simulink model "gm_psk_demodulate_block_fil"  (R2020a)
settings: Solver=FixedStepDiscrete  StartTime=0.0  StopTime=10.0  RelTol=1e-3
libraries: simulink x1, hdlmdlgenlib x1, fillib x1
settings Model: Creator=wardo  LastModifiedBy=wardo
settings DataIOCC: LimitDataPoints=on  SaveOutput=off  SaveTime=off
settings OptimizationCC: BlockReduction=off  ConditionallyExecuteInputs=off  DefaultParameterBehavior=Inlined  LifeSpan=inf
settings DebuggingCC: AlgebraicLoopMsg=error  InheritedTsInSrcMsg=none  SingleTaskRateTransMsg=error  AllowSymbolicDim=off  StrictBusMsg=ErrorOnBusTreatedAsVector  SFUnexpectedBacktrackingDiag=warning  SFNoUnconditionalDefaultTransitionDiag=warning  SFExecutionAtInitializationDiag=none  ArithmeticOperatorsInVariantConditions=warning
settings HardwareCC: ProdBitPerPointer=32  ProdBitPerSizeT=32  ProdBitPerPtrDiffT=32  ProdLargestAtomicFloat=None  ProdIntDivRoundTo=Undefined  ProdEndianess=Unspecified  ProdWordSize=32  ProdHWDeviceType=ASIC/FPGA->ASIC/FPGA  ProdEqTarget=off
settings SFSimCC: SimUseLocalCustomCode=off  CustomCodeUndefinedFunction=UseInterfaceOnly
settings RTWCC: RTWUseLocalCustomCode=off
settings CodeAppCC: StateflowObjectComments=on
settings GRTTargetCC: TargetLangStandard=C89/C90 (ANSI)
settings ConfigComp: CovScope=ReferencedModels  CovMetricSettings=dw  CovHtmlReporting=on  CovSaveCumulativeToWorkspaceVar=on  CovSaveSingleToWorkspaceVar=on  CovExternalEMLEnable=off  CovSFcnEnable=off

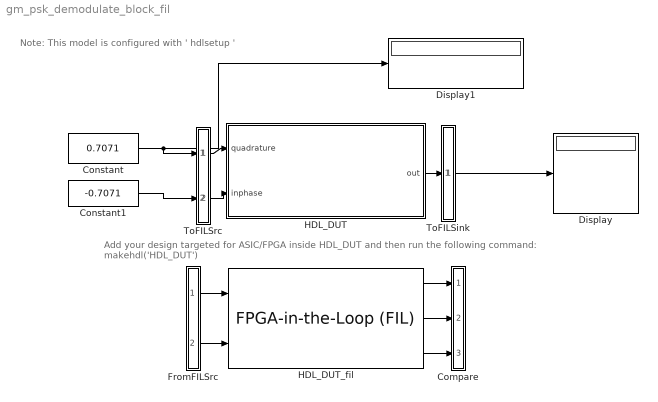
== system gm_psk_demodulate_block_fil ==
  note: Note: This model is configured with ' hdlsetup '
  note: Add your design targeted for ASIC/FPGA inside HDL_DUT and then run the following command:
      | makehdl('HDL_DUT')
  Compare : Subsystem
      mask Display: disp('')
  Constant : Constant  Value=0.7071  OutDataTypeStr=single  SampleTime=-1
  Constant1 : Constant  Value=-0.7071  OutDataTypeStr=single  SampleTime=-1
  Display : Display
  Display1 : Display
  FromFILSrc : Subsystem
      mask Display: disp('')
  HDL_DUT : Subsystem
  HDL_DUT_fil : fillib/FPGA-in-the-Loop (FIL)  ForceInterfaceUpdate=0.90579
      settings: SourceProductBaseCode=ES,HD
  ToFILSink : Subsystem
      mask Display: disp('')
  ToFILSrc : Subsystem
      mask Display: disp('')
  wires:
  Constant/1 -> Display1/1, ToFILSrc/1(in1)
  ToFILSrc/1(out1) -> HDL_DUT/1(quadrature)
  ToFILSrc/2(out2) -> HDL_DUT/2(inphase)
  HDL_DUT/1(out) -> ToFILSink/1(in1)
  Constant1/1 -> ToFILSrc/2(in2)
  ToFILSink/1(out1) -> Display/1
  FromFILSrc/1(out1) -> HDL_DUT_fil/1
  FromFILSrc/2(out2) -> HDL_DUT_fil/2
  HDL_DUT_fil/1 -> Compare/1(in1)
  HDL_DUT_fil/2 -> Compare/2(in2)
  HDL_DUT_fil/3 -> Compare/3(in3)

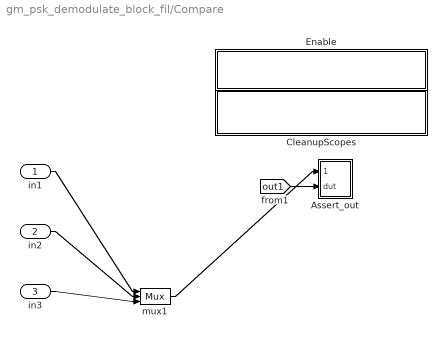
== system gm_psk_demodulate_block_fil/Compare ==
  in1 : Inport
  in2 : Inport  Port=2
  in3 : Inport  Port=3
  Assert_out : Subsystem  mask{ToleranceValue=1e-07}
  CleanupScopes : Subsystem
      settings: OpenFcn=|
      | blkName = gcb; %self block
      | idx = regexp(blkName, '/CleanupScopes$', 'once');
      | blkParent = blkName(1:idx-1);
      | blks=find_system(blkParent, 'LookUnderMasks', 'all','blocktype', 'Scope');
      | for itr = 1:length(blks)
      | 	 hScopeCfg = get_param(blks{itr},'ScopeConfiguration');
      | 	 hScopeCfg.Visible = ~ hScopeCfg.Visible;
      | end
      | drawnow;
      mask Display: fprintf(message('hdlcoder:cosim:vnl_dblclick').getString());
  Enable : Subsystem
      settings: OpenFcn=|
      | blkName = gcb;
      | idx = regexp(blkName, '/Enable$', 'once');
      | blkParent = blkName(1:idx-1);
      | blks=find_system(blkParent, 'LookUnderMasks', 'all','blocktype', 'Assertion');
      | e = get_param(blks{1}, 'Enabled');
      | if strcmp(e, 'on'), f= 'off';, else, f = 'on';, end
      | for ii=1:length(blks), set_param(blks{ii}, 'Enabled', f);, end
      | set_param(gcb, 'MaskDisplay',['fprintf(message(''hdlcoder:cosim:vnl_dblclick_assertions'',','''',upper(e),'''',').getString())']);
      mask Display: fprintf(message('hdlcoder:cosim:vnl_dblclick_assertions','OFF').getString());
  mux1 : Mux  Inputs=3
  wires:
  in3/1 -> mux1/3
  in2/1 -> mux1/2
  in1/1 -> mux1/1
  mux1/1 -> Assert_out/1(cosim)
  [out1] -> Assert_out/2(dut)

== system gm_psk_demodulate_block_fil/FromFILSrc ==
  dtc1 : DataTypeConversion  OutDataTypeStr=single  SaturateOnIntegerOverflow=on  RndMeth=Zero
  dtc2 : DataTypeConversion  OutDataTypeStr=single  SaturateOnIntegerOverflow=on  RndMeth=Zero
  out1 : Outport
  out2 : Outport  Port=2
  wires:
  [in1] -> dtc1/1
  [in2] -> dtc2/1
  dtc1/1 -> out1/1
  dtc2/1 -> out2/1

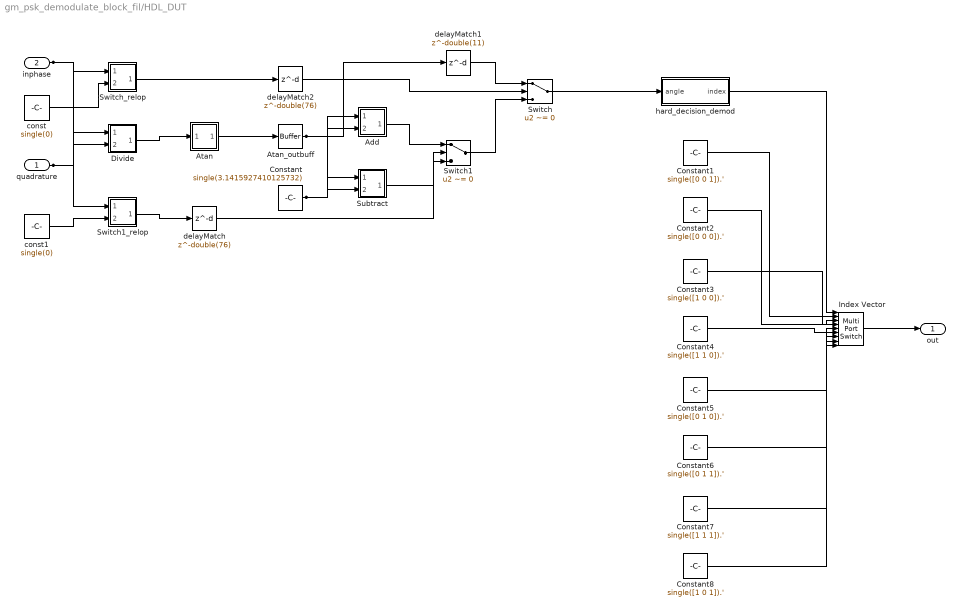
== system gm_psk_demodulate_block_fil/HDL_DUT ==
  quadrature : Inport  OutDataTypeStr=single  PortDimensions=1  SampleTime=0.2
  inphase : Inport  Port=2  OutDataTypeStr=single  PortDimensions=1  SampleTime=0.2
  Add : Subsystem
      mask Display: disp('NFP\nadd');
  Atan : Subsystem
      mask Display: disp('NFP\ntrig');
  Atan_outbuff : hdlmdlgenlib/Buffer
      settings: SourceProductBaseCode=SL
  Constant : Constant  Value=single(3.1415927410125732)  OutDataTypeStr=single  SampleTime=0.2
  Constant1 : Constant  Value=single([0 0 1]).'  OutDataTypeStr=single  SampleTime=0.2
  Constant2 : Constant  Value=single([0 0 0]).'  OutDataTypeStr=single  SampleTime=0.2
  Constant3 : Constant  Value=single([1 0 0]).'  OutDataTypeStr=single  SampleTime=0.2
  Constant4 : Constant  Value=single([1 1 0]).'  OutDataTypeStr=single  SampleTime=0.2
  Constant5 : Constant  Value=single([0 1 0]).'  OutDataTypeStr=single  SampleTime=0.2
  Constant6 : Constant  Value=single([0 1 1]).'  OutDataTypeStr=single  SampleTime=0.2
  Constant7 : Constant  Value=single([1 1 1]).'  OutDataTypeStr=single  SampleTime=0.2
  Constant8 : Constant  Value=single([1 0 1]).'  OutDataTypeStr=single  SampleTime=0.2
  Divide : Subsystem
      mask Display: disp('NFP\nmul');
  Index Vector : MultiPortSwitch  Inputs=8  DiagnosticForDefault=None  OutDataTypeStr=single  SampleTime=0.2
  Subtract : Subsystem
      mask Display: disp('NFP\nadd');
  Switch : Switch  Criteria=u2 ~= 0  Threshold=double(0)  OutDataTypeStr=single  SampleTime=0.2
  Switch1 : Switch  Criteria=u2 ~= 0  Threshold=double(0)  OutDataTypeStr=single  SampleTime=0.2
  Switch1_relop : Subsystem
      mask Display: disp('NFP\nrelop');
  Switch_relop : Subsystem
      mask Display: disp('NFP\nrelop');
  const : Constant  Value=single(0)  OutDataTypeStr=single  SampleTime=0.2
  const1 : Constant  Value=single(0)  OutDataTypeStr=single  SampleTime=0.2
  delayMatch : Delay  DelayLength=double(76)  InitialCondition=0  SampleTime=0.2
  delayMatch1 : Delay  DelayLength=double(11)  InitialCondition=0  SampleTime=0.2
  delayMatch2 : Delay  DelayLength=double(76)  InitialCondition=0  SampleTime=0.2
  hard_decision_demod : Subsystem
  out : Outport  VectorParamsAs1DForOutWhenUnconnected=off
  wires:
  Atan_outbuff/1 -> Add/2(In2), Subtract/1(In1), delayMatch1/1
  Switch1_relop/1(Out1) -> delayMatch/1
  Switch_relop/1(Out1) -> delayMatch2/1
  Subtract/1(Out1) -> Switch1/3
  Divide/1(Out1) -> Atan/1(In1)
  Atan/1(Out1) -> Atan_outbuff/1
  Add/1(Out1) -> Switch1/1
  delayMatch/1 -> Switch1/2
  const1/1 -> Switch1_relop/2(In2)
  delayMatch2/1 -> Switch/2
  const/1 -> Switch_relop/2(In2)
  hard_decision_demod/1(index) -> Index Vector/1
  Switch1/1 -> Switch/3
  Switch/1 -> hard_decision_demod/1(angle)
  Index Vector/1 -> out/1
  Constant8/1 -> Index Vector/9
  Constant7/1 -> Index Vector/8
  Constant6/1 -> Index Vector/7
  Constant5/1 -> Index Vector/6
  Constant4/1 -> Index Vector/5
  Constant3/1 -> Index Vector/4
  Constant2/1 -> Index Vector/3
  Constant1/1 -> Index Vector/2
  Constant/1 -> Add/1(In1), Subtract/2(In2)
  delayMatch1/1 -> Switch/1
  inphase/1 -> Divide/2(In2), Switch_relop/1(In1)
  quadrature/1 -> Divide/1(In1), Switch1_relop/1(In1)

== system gm_psk_demodulate_block_fil/ToFILSink ==
  in1 : Inport
  out1 : Outport
  tag scope: out1=global
  wires:
  in1/1 -> out1/1, [out1]

== system gm_psk_demodulate_block_fil/ToFILSrc ==
  in1 : Inport
  in2 : Inport  Port=2
  out1 : Outport
  out2 : Outport  Port=2
  tag scope: in1=global, in2=global
  wires:
  in1/1 -> out1/1, [in1]
  in2/1 -> out2/1, [in2]

== system gm_psk_demodulate_block_fil/Compare/Assert_out ==
  cosim : Inport
  dut : Inport  Port=2
  AssertEq : Assertion  StopWhenAssertionFail=off
  Compare To Zero : simulink/Logic and Bit Operations/Compare To Zero  relop===  OutDataTypeStr=boolean
  RelErrCheck : Subsystem
  compare: out : Scope  NumInputPorts=3
  wires:
  dut/1 -> compare: out/2, RelErrCheck/2(In2)  "dut ref"
  cosim/1 -> compare: out/1, RelErrCheck/1(In1)  "cosim"
  RelErrCheck/1(Out1) -> AssertEq/1, Compare To Zero/1
  Compare To Zero/1 -> compare: out/3  "err"

== system gm_psk_demodulate_block_fil/Compare/CleanupScopes ==

== system gm_psk_demodulate_block_fil/Compare/Enable ==

== system gm_psk_demodulate_block_fil/HDL_DUT/Add ==
  In1 : Inport
  In2 : Inport  Port=2
  Add : Sum  OutDataTypeStr=single  SampleTime=0.2
  Add_pd1 : Delay  DelayLength=11
  Out1 : Outport
  wires:
  Add_pd1/1 -> Out1/1
  Add/1 -> Add_pd1/1
  In2/1 -> Add/2
  In1/1 -> Add/1

== system gm_psk_demodulate_block_fil/HDL_DUT/Atan ==
  In1 : Inport
  Atan : Trigonometry  Operator=atan  SampleTime=0.2
  Atan_pd1 : Delay  DelayLength=36
  Out1 : Outport
  wires:
  Atan_pd1/1 -> Out1/1
  Atan/1 -> Atan_pd1/1
  In1/1 -> Atan/1

== system gm_psk_demodulate_block_fil/HDL_DUT/Divide ==
  In1 : Inport
  In2 : Inport  Port=2
  Divide : Product  Inputs=*/  OutDataTypeStr=single  SaturateOnIntegerOverflow=on  SampleTime=0.2
  Divide_pd1 : Delay  DelayLength=32
  Out1 : Outport
  wires:
  Divide_pd1/1 -> Out1/1
  Divide/1 -> Divide_pd1/1
  In2/1 -> Divide/2
  In1/1 -> Divide/1

== system gm_psk_demodulate_block_fil/HDL_DUT/Subtract ==
  In1 : Inport
  In2 : Inport  Port=2
  Subtract : Sum  Inputs=+-  OutDataTypeStr=single  SampleTime=0.2
  Subtract_pd1 : Delay  DelayLength=11
  Out1 : Outport
  wires:
  Subtract_pd1/1 -> Out1/1
  Subtract/1 -> Subtract_pd1/1
  In2/1 -> Subtract/2
  In1/1 -> Subtract/1

== system gm_psk_demodulate_block_fil/HDL_DUT/Switch1_relop ==
  In1 : Inport
  In2 : Inport  Port=2
  Switch1_relop : RelationalOperator  OutDataTypeStr=boolean  SampleTime=0.2  RndMeth=Nearest
  Switch1_relop_pd1 : Delay  DelayLength=3
  Out1 : Outport
  wires:
  Switch1_relop_pd1/1 -> Out1/1
  Switch1_relop/1 -> Switch1_relop_pd1/1
  In2/1 -> Switch1_relop/2
  In1/1 -> Switch1_relop/1

== system gm_psk_demodulate_block_fil/HDL_DUT/Switch_relop ==
  In1 : Inport
  In2 : Inport  Port=2
  Switch_relop : RelationalOperator  OutDataTypeStr=boolean  SampleTime=0.2  RndMeth=Nearest
  Switch_relop_pd1 : Delay  DelayLength=3
  Out1 : Outport
  wires:
  Switch_relop_pd1/1 -> Out1/1
  Switch_relop/1 -> Switch_relop_pd1/1
  In2/1 -> Switch_relop/2
  In1/1 -> Switch_relop/1

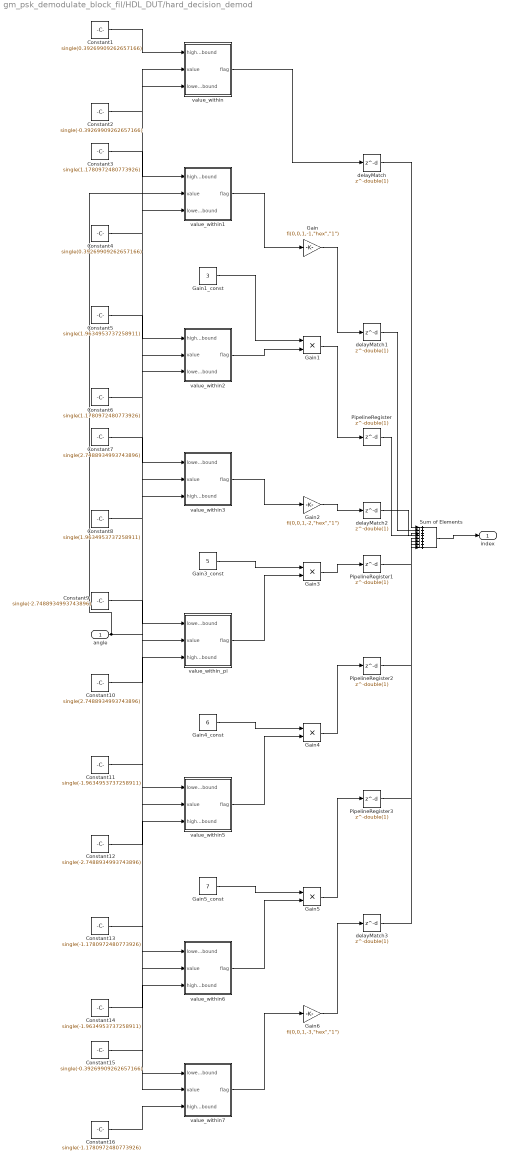
== system gm_psk_demodulate_block_fil/HDL_DUT/hard_decision_demod ==
  angle : Inport  OutDataTypeStr=single  PortDimensions=1  SampleTime=0.2
  Constant1 : Constant  Value=single(0.39269909262657166)  OutDataTypeStr=single  SampleTime=0.2
  Constant10 : Constant  Value=single(2.7488934993743896)  OutDataTypeStr=single  SampleTime=0.2
  Constant11 : Constant  Value=single(-1.9634953737258911)  OutDataTypeStr=single  SampleTime=0.2
  Constant12 : Constant  Value=single(-2.7488934993743896)  OutDataTypeStr=single  SampleTime=0.2
  Constant13 : Constant  Value=single(-1.1780972480773926)  OutDataTypeStr=single  SampleTime=0.2
  Constant14 : Constant  Value=single(-1.9634953737258911)  OutDataTypeStr=single  SampleTime=0.2
  Constant15 : Constant  Value=single(-0.39269909262657166)  OutDataTypeStr=single  SampleTime=0.2
  Constant16 : Constant  Value=single(-1.1780972480773926)  OutDataTypeStr=single  SampleTime=0.2
  Constant2 : Constant  Value=single(-0.39269909262657166)  OutDataTypeStr=single  SampleTime=0.2
  Constant3 : Constant  Value=single(1.1780972480773926)  OutDataTypeStr=single  SampleTime=0.2
  Constant4 : Constant  Value=single(0.39269909262657166)  OutDataTypeStr=single  SampleTime=0.2
  Constant5 : Constant  Value=single(1.9634953737258911)  OutDataTypeStr=single  SampleTime=0.2
  Constant6 : Constant  Value=single(1.1780972480773926)  OutDataTypeStr=single  SampleTime=0.2
  Constant7 : Constant  Value=single(2.7488934993743896)  OutDataTypeStr=single  SampleTime=0.2
  Constant8 : Constant  Value=single(1.9634953737258911)  OutDataTypeStr=single  SampleTime=0.2
  Constant9 : Constant  Value=single(-2.7488934993743896)  OutDataTypeStr=single  SampleTime=0.2
  Gain : Gain  Gain="fi(0,0,1,-1,\"hex\",\"1\")"  ParamDataTypeStr=fixdt(0, 1, -1)  OutDataTypeStr=fixdt(0, 1, -1)  SampleTime=0.2
  Gain1 : Product  Inputs=**  OutDataTypeStr=fixdt(0, 2, 0)  SampleTime=0.2
  Gain1_const : Constant  Value=3  OutDataTypeStr=fixdt(0, 2, 0)  SampleTime=0.2
  Gain2 : Gain  Gain="fi(0,0,1,-2,\"hex\",\"1\")"  ParamDataTypeStr=fixdt(0, 1, -2)  OutDataTypeStr=fixdt(0, 1, -2)  SampleTime=0.2
  Gain3 : Product  Inputs=**  OutDataTypeStr=fixdt(0, 3, 0)  SampleTime=0.2
  Gain3_const : Constant  Value=5  OutDataTypeStr=fixdt(0, 3, 0)  SampleTime=0.2
  Gain4 : Product  Inputs=**  OutDataTypeStr=fixdt(0, 2, -1)  SampleTime=0.2
  Gain4_const : Constant  Value=6  OutDataTypeStr=fixdt(0, 2, -1)  SampleTime=0.2
  Gain5 : Product  Inputs=**  OutDataTypeStr=fixdt(0, 3, 0)  SampleTime=0.2
  Gain5_const : Constant  Value=7  OutDataTypeStr=fixdt(0, 3, 0)  SampleTime=0.2
  Gain6 : Gain  Gain="fi(0,0,1,-3,\"hex\",\"1\")"  ParamDataTypeStr=fixdt(0, 1, -3)  OutDataTypeStr=fixdt(0, 1, -3)  SampleTime=0.2
  PipelineRegister{,1..3} (4 alike) : Delay  DelayLength=double(1)  InitialCondition=0  SampleTime=0.2
  Sum of Elements : Sum  Inputs=++++++++  AccumDataTypeStr=fixdt(0, 9, 0)  OutDataTypeStr=fixdt(0, 9, 0)  SampleTime=0.2
  delayMatch{,1..3} (4 alike) : Delay  DelayLength=double(1)  InitialCondition=0  SampleTime=0.2
  value_within : Subsystem
  value_within1 : Subsystem
  value_within2 : Subsystem
  value_within3 : Subsystem
  value_within5 : Subsystem
  value_within6 : Subsystem
  value_within7 : Subsystem
  value_within_pi : Subsystem
  index : Outport
  wires:
  Gain5/1 -> PipelineRegister3/1
  Gain4/1 -> PipelineRegister2/1
  Gain3/1 -> PipelineRegister1/1
  Gain1/1 -> PipelineRegister/1
  angle/1 -> value_within_pi/2(value), value_within5/2(value), value_within6/2(value), value_within7/2(value), value_within3/2(value), value_within2/2(value), value_within/2(value), value_within1/2(value)
  Gain6/1 -> delayMatch3/1
  Gain2/1 -> delayMatch2/1
  Gain/1 -> delayMatch1/1
  value_within/1(flag) -> delayMatch/1
  Gain5_const/1 -> Gain5/1
  Gain4_const/1 -> Gain4/1
  Gain3_const/1 -> Gain3/1
  Gain1_const/1 -> Gain1/1
  value_within_pi/1(flag) -> Gain3/2
  value_within7/1(flag) -> Gain6/1
  value_within6/1(flag) -> Gain5/2
  value_within5/1(flag) -> Gain4/2
  value_within3/1(flag) -> Gain2/1
  value_within2/1(flag) -> Gain1/2
  value_within1/1(flag) -> Gain/1
  delayMatch/1 -> Sum of Elements/1
  Sum of Elements/1 -> index/1
  delayMatch3/1 -> Sum of Elements/8
  PipelineRegister3/1 -> Sum of Elements/7
  PipelineRegister2/1 -> Sum of Elements/6
  PipelineRegister1/1 -> Sum of Elements/5
  delayMatch2/1 -> Sum of Elements/4
  PipelineRegister/1 -> Sum of Elements/3
  delayMatch1/1 -> Sum of Elements/2
  Constant9/1 -> value_within_pi/1(lower_bound)
  Constant8/1 -> value_within3/3(higher_bound)
  Constant7/1 -> value_within3/1(lower_bound)
  Constant6/1 -> value_within2/3(lower_bound)
  Constant5/1 -> value_within2/1(higher_bound)
  Constant4/1 -> value_within1/3(lower_bound)
  Constant3/1 -> value_within1/1(higher_bound)
  Constant2/1 -> value_within/3(lower_bound)
  Constant16/1 -> value_within7/3(higher_bound)
  Constant15/1 -> value_within7/1(lower_bound)
  Constant14/1 -> value_within6/3(higher_bound)
  Constant13/1 -> value_within6/1(lower_bound)
  Constant12/1 -> value_within5/3(higher_bound)
  Constant11/1 -> value_within5/1(lower_bound)
  Constant10/1 -> value_within_pi/3(higher_bound)
  Constant1/1 -> value_within/1(higher_bound)

== system gm_psk_demodulate_block_fil/Compare/Assert_out/RelErrCheck ==
  In1 : Inport
  In2 : Inport  Port=2
  "RelativeErrorCheck " : MATLAB Function  TreatAsAtomicUnit=on
  Out1 : Outport  VectorParamsAs1DForOutWhenUnconnected=off
  wires:
  In2/1 -> "RelativeErrorCheck "/2(R)
  In1/1 -> "RelativeErrorCheck "/1(P)
  "RelativeErrorCheck "/1(y) -> Out1/1

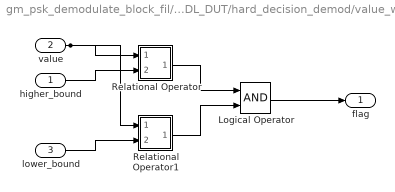
== system gm_psk_demodulate_block_fil/HDL_DUT/hard_decision_demod/value_within ==
  higher_bound : Inport  OutDataTypeStr=single  PortDimensions=1  SampleTime=0.2
  value : Inport  Port=2  OutDataTypeStr=single  PortDimensions=1  SampleTime=0.2
  lower_bound : Inport  Port=3  OutDataTypeStr=single  PortDimensions=1  SampleTime=0.2
  Logical Operator : Logic  AllPortsSameDT=off  OutDataTypeStr=boolean  SampleTime=0.2
  Relational Operator : Subsystem
      mask Display: disp('NFP\nrelop');
  Relational Operator1 : Subsystem
      mask Display: disp('NFP\nrelop');
  flag : Outport
  wires:
  lower_bound/1 -> Relational Operator1/2(In2)
  value/1 -> Relational Operator/1(In1), Relational Operator1/1(In1)
  higher_bound/1 -> Relational Operator/2(In2)
  Relational Operator1/1(Out1) -> Logical Operator/2
  Relational Operator/1(Out1) -> Logical Operator/1
  Logical Operator/1 -> flag/1

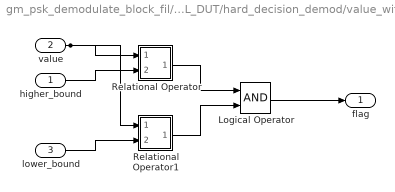
== system gm_psk_demodulate_block_fil/HDL_DUT/hard_decision_demod/value_within1 ==
  higher_bound : Inport  OutDataTypeStr=single  PortDimensions=1  SampleTime=0.2
  value : Inport  Port=2  OutDataTypeStr=single  PortDimensions=1  SampleTime=0.2
  lower_bound : Inport  Port=3  OutDataTypeStr=single  PortDimensions=1  SampleTime=0.2
  Logical Operator : Logic  AllPortsSameDT=off  OutDataTypeStr=boolean  SampleTime=0.2
  Relational Operator : Subsystem
      mask Display: disp('NFP\nrelop');
  Relational Operator1 : Subsystem
      mask Display: disp('NFP\nrelop');
  flag : Outport
  wires:
  Logical Operator/1 -> flag/1
  Relational Operator/1(Out1) -> Logical Operator/1
  Relational Operator1/1(Out1) -> Logical Operator/2
  higher_bound/1 -> Relational Operator/2(In2)
  value/1 -> Relational Operator1/1(In1), Relational Operator/1(In1)
  lower_bound/1 -> Relational Operator1/2(In2)

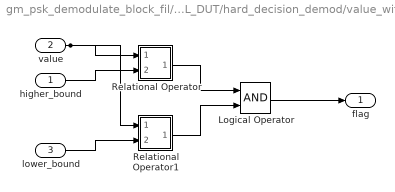
== system gm_psk_demodulate_block_fil/HDL_DUT/hard_decision_demod/value_within2 ==
  higher_bound : Inport  OutDataTypeStr=single  PortDimensions=1  SampleTime=0.2
  value : Inport  Port=2  OutDataTypeStr=single  PortDimensions=1  SampleTime=0.2
  lower_bound : Inport  Port=3  OutDataTypeStr=single  PortDimensions=1  SampleTime=0.2
  Logical Operator : Logic  AllPortsSameDT=off  OutDataTypeStr=boolean  SampleTime=0.2
  Relational Operator : Subsystem
      mask Display: disp('NFP\nrelop');
  Relational Operator1 : Subsystem
      mask Display: disp('NFP\nrelop');
  flag : Outport
  wires:
  Logical Operator/1 -> flag/1
  Relational Operator/1(Out1) -> Logical Operator/1
  Relational Operator1/1(Out1) -> Logical Operator/2
  higher_bound/1 -> Relational Operator/2(In2)
  value/1 -> Relational Operator1/1(In1), Relational Operator/1(In1)
  lower_bound/1 -> Relational Operator1/2(In2)

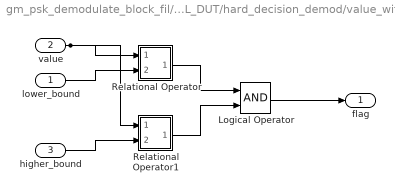
== system gm_psk_demodulate_block_fil/HDL_DUT/hard_decision_demod/value_within3 ==
  lower_bound : Inport  OutDataTypeStr=single  PortDimensions=1  SampleTime=0.2
  value : Inport  Port=2  OutDataTypeStr=single  PortDimensions=1  SampleTime=0.2
  higher_bound : Inport  Port=3  OutDataTypeStr=single  PortDimensions=1  SampleTime=0.2
  Logical Operator : Logic  AllPortsSameDT=off  OutDataTypeStr=boolean  SampleTime=0.2
  Relational Operator : Subsystem
      mask Display: disp('NFP\nrelop');
  Relational Operator1 : Subsystem
      mask Display: disp('NFP\nrelop');
  flag : Outport
  wires:
  higher_bound/1 -> Relational Operator1/2(In2)
  value/1 -> Relational Operator/1(In1), Relational Operator1/1(In1)
  lower_bound/1 -> Relational Operator/2(In2)
  Relational Operator1/1(Out1) -> Logical Operator/2
  Relational Operator/1(Out1) -> Logical Operator/1
  Logical Operator/1 -> flag/1

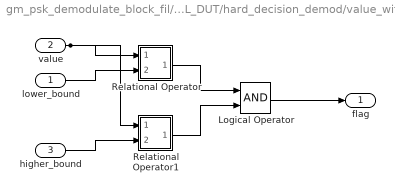
== system gm_psk_demodulate_block_fil/HDL_DUT/hard_decision_demod/value_within5 ==
  lower_bound : Inport  OutDataTypeStr=single  PortDimensions=1  SampleTime=0.2
  value : Inport  Port=2  OutDataTypeStr=single  PortDimensions=1  SampleTime=0.2
  higher_bound : Inport  Port=3  OutDataTypeStr=single  PortDimensions=1  SampleTime=0.2
  Logical Operator : Logic  AllPortsSameDT=off  OutDataTypeStr=boolean  SampleTime=0.2
  Relational Operator : Subsystem
      mask Display: disp('NFP\nrelop');
  Relational Operator1 : Subsystem
      mask Display: disp('NFP\nrelop');
  flag : Outport
  wires:
  higher_bound/1 -> Relational Operator1/2(In2)
  value/1 -> Relational Operator/1(In1), Relational Operator1/1(In1)
  lower_bound/1 -> Relational Operator/2(In2)
  Relational Operator1/1(Out1) -> Logical Operator/2
  Relational Operator/1(Out1) -> Logical Operator/1
  Logical Operator/1 -> flag/1

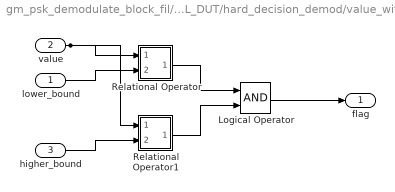
== system gm_psk_demodulate_block_fil/HDL_DUT/hard_decision_demod/value_within6 ==
  lower_bound : Inport  OutDataTypeStr=single  PortDimensions=1  SampleTime=0.2
  value : Inport  Port=2  OutDataTypeStr=single  PortDimensions=1  SampleTime=0.2
  higher_bound : Inport  Port=3  OutDataTypeStr=single  PortDimensions=1  SampleTime=0.2
  Logical Operator : Logic  AllPortsSameDT=off  OutDataTypeStr=boolean  SampleTime=0.2
  Relational Operator : Subsystem
      mask Display: disp('NFP\nrelop');
  Relational Operator1 : Subsystem
      mask Display: disp('NFP\nrelop');
  flag : Outport
  wires:
  Logical Operator/1 -> flag/1
  Relational Operator/1(Out1) -> Logical Operator/1
  Relational Operator1/1(Out1) -> Logical Operator/2
  lower_bound/1 -> Relational Operator/2(In2)
  value/1 -> Relational Operator1/1(In1), Relational Operator/1(In1)
  higher_bound/1 -> Relational Operator1/2(In2)

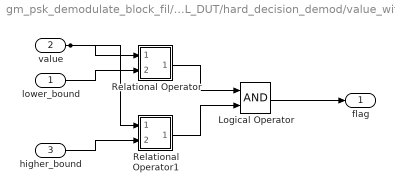
== system gm_psk_demodulate_block_fil/HDL_DUT/hard_decision_demod/value_within7 ==
  lower_bound : Inport  OutDataTypeStr=single  PortDimensions=1  SampleTime=0.2
  value : Inport  Port=2  OutDataTypeStr=single  PortDimensions=1  SampleTime=0.2
  higher_bound : Inport  Port=3  OutDataTypeStr=single  PortDimensions=1  SampleTime=0.2
  Logical Operator : Logic  AllPortsSameDT=off  OutDataTypeStr=boolean  SampleTime=0.2
  Relational Operator : Subsystem
      mask Display: disp('NFP\nrelop');
  Relational Operator1 : Subsystem
      mask Display: disp('NFP\nrelop');
  flag : Outport
  wires:
  Logical Operator/1 -> flag/1
  Relational Operator/1(Out1) -> Logical Operator/1
  Relational Operator1/1(Out1) -> Logical Operator/2
  lower_bound/1 -> Relational Operator/2(In2)
  value/1 -> Relational Operator1/1(In1), Relational Operator/1(In1)
  higher_bound/1 -> Relational Operator1/2(In2)

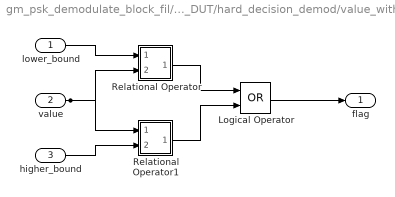
== system gm_psk_demodulate_block_fil/HDL_DUT/hard_decision_demod/value_within_pi ==
  lower_bound : Inport  OutDataTypeStr=single  PortDimensions=1  SampleTime=0.2
  value : Inport  Port=2  OutDataTypeStr=single  PortDimensions=1  SampleTime=0.2
  higher_bound : Inport  Port=3  OutDataTypeStr=single  PortDimensions=1  SampleTime=0.2
  Logical Operator : Logic  Operator=OR  AllPortsSameDT=off  OutDataTypeStr=boolean  SampleTime=0.2
  Relational Operator : Subsystem
      mask Display: disp('NFP\nrelop');
  Relational Operator1 : Subsystem
      mask Display: disp('NFP\nrelop');
  flag : Outport
  wires:
  higher_bound/1 -> Relational Operator1/2(In2)
  value/1 -> Relational Operator/2(In2), Relational Operator1/1(In1)
  lower_bound/1 -> Relational Operator/1(In1)
  Relational Operator1/1(Out1) -> Logical Operator/2
  Relational Operator/1(Out1) -> Logical Operator/1
  Logical Operator/1 -> flag/1

== system gm_psk_demodulate_block_fil/HDL_DUT/hard_decision_demod/value_within/Relational Operator ==
  In1 : Inport
  In2 : Inport  Port=2
  Relational Operator : RelationalOperator  Operator=<  OutDataTypeStr=boolean  SampleTime=0.2  RndMeth=Nearest
  Relational Operator_pd1 : Delay  DelayLength=3
  Out1 : Outport
  wires:
  Relational Operator_pd1/1 -> Out1/1
  Relational Operator/1 -> Relational Operator_pd1/1
  In2/1 -> Relational Operator/2
  In1/1 -> Relational Operator/1

== system gm_psk_demodulate_block_fil/HDL_DUT/hard_decision_demod/value_within/Relational Operator1 ==
  In1 : Inport
  In2 : Inport  Port=2
  Relational Operator1 : RelationalOperator  OutDataTypeStr=boolean  SampleTime=0.2  RndMeth=Nearest
  Relational Operator1_pd1 : Delay  DelayLength=3
  Out1 : Outport
  wires:
  Relational Operator1_pd1/1 -> Out1/1
  Relational Operator1/1 -> Relational Operator1_pd1/1
  In2/1 -> Relational Operator1/2
  In1/1 -> Relational Operator1/1

== system gm_psk_demodulate_block_fil/HDL_DUT/hard_decision_demod/value_within1/Relational Operator ==
  In1 : Inport
  In2 : Inport  Port=2
  Relational Operator : RelationalOperator  Operator=<  OutDataTypeStr=boolean  SampleTime=0.2  RndMeth=Nearest
  Relational Operator_pd1 : Delay  DelayLength=3
  Out1 : Outport
  wires:
  In1/1 -> Relational Operator/1
  In2/1 -> Relational Operator/2
  Relational Operator/1 -> Relational Operator_pd1/1
  Relational Operator_pd1/1 -> Out1/1

== system gm_psk_demodulate_block_fil/HDL_DUT/hard_decision_demod/value_within1/Relational Operator1 ==
  In1 : Inport
  In2 : Inport  Port=2
  Relational Operator1 : RelationalOperator  OutDataTypeStr=boolean  SampleTime=0.2  RndMeth=Nearest
  Relational Operator1_pd1 : Delay  DelayLength=3
  Out1 : Outport
  wires:
  In1/1 -> Relational Operator1/1
  In2/1 -> Relational Operator1/2
  Relational Operator1/1 -> Relational Operator1_pd1/1
  Relational Operator1_pd1/1 -> Out1/1

== system gm_psk_demodulate_block_fil/HDL_DUT/hard_decision_demod/value_within2/Relational Operator ==
  In1 : Inport
  In2 : Inport  Port=2
  Relational Operator : RelationalOperator  Operator=<  OutDataTypeStr=boolean  SampleTime=0.2  RndMeth=Nearest
  Relational Operator_pd1 : Delay  DelayLength=3
  Out1 : Outport
  wires:
  In1/1 -> Relational Operator/1
  In2/1 -> Relational Operator/2
  Relational Operator/1 -> Relational Operator_pd1/1
  Relational Operator_pd1/1 -> Out1/1

== system gm_psk_demodulate_block_fil/HDL_DUT/hard_decision_demod/value_within2/Relational Operator1 ==
  In1 : Inport
  In2 : Inport  Port=2
  Relational Operator1 : RelationalOperator  OutDataTypeStr=boolean  SampleTime=0.2  RndMeth=Nearest
  Relational Operator1_pd1 : Delay  DelayLength=3
  Out1 : Outport
  wires:
  In1/1 -> Relational Operator1/1
  In2/1 -> Relational Operator1/2
  Relational Operator1/1 -> Relational Operator1_pd1/1
  Relational Operator1_pd1/1 -> Out1/1

== system gm_psk_demodulate_block_fil/HDL_DUT/hard_decision_demod/value_within3/Relational Operator ==
  In1 : Inport
  In2 : Inport  Port=2
  Relational Operator : RelationalOperator  Operator=<  OutDataTypeStr=boolean  SampleTime=0.2  RndMeth=Nearest
  Relational Operator_pd1 : Delay  DelayLength=3
  Out1 : Outport
  wires:
  Relational Operator_pd1/1 -> Out1/1
  Relational Operator/1 -> Relational Operator_pd1/1
  In2/1 -> Relational Operator/2
  In1/1 -> Relational Operator/1

== system gm_psk_demodulate_block_fil/HDL_DUT/hard_decision_demod/value_within3/Relational Operator1 ==
  In1 : Inport
  In2 : Inport  Port=2
  Relational Operator1 : RelationalOperator  OutDataTypeStr=boolean  SampleTime=0.2  RndMeth=Nearest
  Relational Operator1_pd1 : Delay  DelayLength=3
  Out1 : Outport
  wires:
  Relational Operator1_pd1/1 -> Out1/1
  Relational Operator1/1 -> Relational Operator1_pd1/1
  In2/1 -> Relational Operator1/2
  In1/1 -> Relational Operator1/1

== system gm_psk_demodulate_block_fil/HDL_DUT/hard_decision_demod/value_within5/Relational Operator ==
  In1 : Inport
  In2 : Inport  Port=2
  Relational Operator : RelationalOperator  Operator=<  OutDataTypeStr=boolean  SampleTime=0.2  RndMeth=Nearest
  Relational Operator_pd1 : Delay  DelayLength=3
  Out1 : Outport
  wires:
  Relational Operator_pd1/1 -> Out1/1
  Relational Operator/1 -> Relational Operator_pd1/1
  In2/1 -> Relational Operator/2
  In1/1 -> Relational Operator/1

== system gm_psk_demodulate_block_fil/HDL_DUT/hard_decision_demod/value_within5/Relational Operator1 ==
  In1 : Inport
  In2 : Inport  Port=2
  Relational Operator1 : RelationalOperator  OutDataTypeStr=boolean  SampleTime=0.2  RndMeth=Nearest
  Relational Operator1_pd1 : Delay  DelayLength=3
  Out1 : Outport
  wires:
  Relational Operator1_pd1/1 -> Out1/1
  Relational Operator1/1 -> Relational Operator1_pd1/1
  In2/1 -> Relational Operator1/2
  In1/1 -> Relational Operator1/1

== system gm_psk_demodulate_block_fil/HDL_DUT/hard_decision_demod/value_within6/Relational Operator ==
  In1 : Inport
  In2 : Inport  Port=2
  Relational Operator : RelationalOperator  Operator=<  OutDataTypeStr=boolean  SampleTime=0.2  RndMeth=Nearest
  Relational Operator_pd1 : Delay  DelayLength=3
  Out1 : Outport
  wires:
  In1/1 -> Relational Operator/1
  In2/1 -> Relational Operator/2
  Relational Operator/1 -> Relational Operator_pd1/1
  Relational Operator_pd1/1 -> Out1/1

== system gm_psk_demodulate_block_fil/HDL_DUT/hard_decision_demod/value_within6/Relational Operator1 ==
  In1 : Inport
  In2 : Inport  Port=2
  Relational Operator1 : RelationalOperator  OutDataTypeStr=boolean  SampleTime=0.2  RndMeth=Nearest
  Relational Operator1_pd1 : Delay  DelayLength=3
  Out1 : Outport
  wires:
  In1/1 -> Relational Operator1/1
  In2/1 -> Relational Operator1/2
  Relational Operator1/1 -> Relational Operator1_pd1/1
  Relational Operator1_pd1/1 -> Out1/1

== system gm_psk_demodulate_block_fil/HDL_DUT/hard_decision_demod/value_within7/Relational Operator ==
  In1 : Inport
  In2 : Inport  Port=2
  Relational Operator : RelationalOperator  Operator=<  OutDataTypeStr=boolean  SampleTime=0.2  RndMeth=Nearest
  Relational Operator_pd1 : Delay  DelayLength=3
  Out1 : Outport
  wires:
  In1/1 -> Relational Operator/1
  In2/1 -> Relational Operator/2
  Relational Operator/1 -> Relational Operator_pd1/1
  Relational Operator_pd1/1 -> Out1/1

== system gm_psk_demodulate_block_fil/HDL_DUT/hard_decision_demod/value_within7/Relational Operator1 ==
  In1 : Inport
  In2 : Inport  Port=2
  Relational Operator1 : RelationalOperator  OutDataTypeStr=boolean  SampleTime=0.2  RndMeth=Nearest
  Relational Operator1_pd1 : Delay  DelayLength=3
  Out1 : Outport
  wires:
  In1/1 -> Relational Operator1/1
  In2/1 -> Relational Operator1/2
  Relational Operator1/1 -> Relational Operator1_pd1/1
  Relational Operator1_pd1/1 -> Out1/1

== system gm_psk_demodulate_block_fil/HDL_DUT/hard_decision_demod/value_within_pi/Relational Operator ==
  In1 : Inport
  In2 : Inport  Port=2
  Relational Operator : RelationalOperator  Operator=>  OutDataTypeStr=boolean  SampleTime=0.2  RndMeth=Nearest
  Relational Operator_pd1 : Delay  DelayLength=3
  Out1 : Outport
  wires:
  Relational Operator_pd1/1 -> Out1/1
  Relational Operator/1 -> Relational Operator_pd1/1
  In2/1 -> Relational Operator/2
  In1/1 -> Relational Operator/1

== system gm_psk_demodulate_block_fil/HDL_DUT/hard_decision_demod/value_within_pi/Relational Operator1 ==
  In1 : Inport
  In2 : Inport  Port=2
  Relational Operator1 : RelationalOperator  OutDataTypeStr=boolean  SampleTime=0.2  RndMeth=Nearest
  Relational Operator1_pd1 : Delay  DelayLength=3
  Out1 : Outport
  wires:
  Relational Operator1_pd1/1 -> Out1/1
  Relational Operator1/1 -> Relational Operator1_pd1/1
  In2/1 -> Relational Operator1/2
  In1/1 -> Relational Operator1/1

== matlab function gm_psk_demodulate_block_fil/Compare/Assert_out/RelErrCheck/RelativeErrorCheck  ==
  data: P input; y output; R input; ToleranceValue parameter double
% Check if the relative error of R with respect to P is below
% ToleranceValue
% P, R are floating-point
function y = relErrCheck(P,R, ToleranceValue)
    tol = ToleranceValue;
    sz = numel(P);
    assert(sz == numel(R), 'Inputs P and R have different sizes.');
    y = false(1, sz);

    for ii=1:sz
        if (isnan(P(ii)) || isnan(R(ii)))
            if (isnan(P(ii)) && isnan(R(ii)))
                y(ii) = true;
            end
        elseif (isinf(P(ii)) || isinf(R(ii)))
            y(ii) = (P(ii) == R(ii));
        elseif (P(ii) == 0)
            y(ii) = (R(ii) == 0);
        else
            absdiff = abs(P(ii) - R(ii));
            relerr = absdiff/abs(P(ii));
            y(ii) = (relerr <= tol);
        end
    end
end
